simulink model "CSE_SIMULINK_BLOCK_DIAGRAM_NO1"  (R2022b)
settings: Solver=VariableStepAuto  StartTime=0.0  StopTime=10  RelTol=1e-3
undefined symbols (not defined in the file): G1_den, G2_den, G3_den, G_num, H1_den, H2_den, H3_den, H_num, tfden, tfnum
settings Model: Creator=tolen  LastModifiedBy=tolen

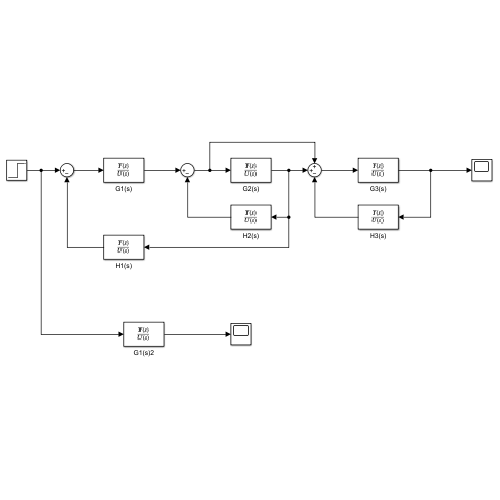
[thumbnail: Simulink's stored preview of the top-level diagram]
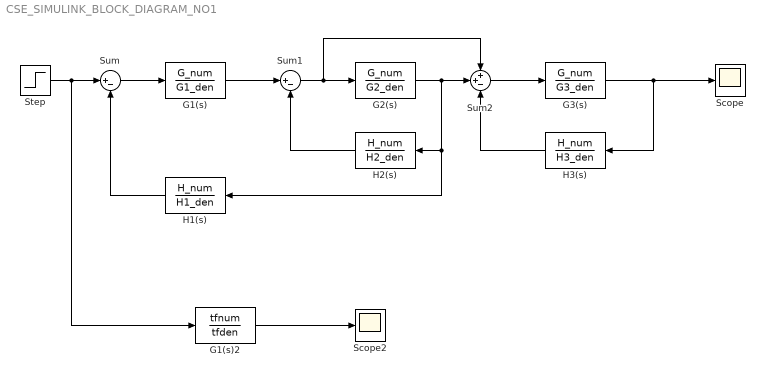
== system CSE_SIMULINK_BLOCK_DIAGRAM_NO1 ==
  G1(s) : TransferFcn  Numerator=G_num  Denominator=G1_den
  G1(s)2 : TransferFcn  Numerator=tfnum  Denominator=tfden
  G2(s) : TransferFcn  Numerator=G_num  Denominator=G2_den
  G3(s) : TransferFcn  Numerator=G_num  Denominator=G3_den
  H1(s) : TransferFcn  Numerator=H_num  Denominator=H1_den
  H2(s) : TransferFcn  Numerator=H_num  Denominator=H2_den
  H3(s) : TransferFcn  Numerator=H_num  Denominator=H3_den
  Scope : Scope
  Scope2 : Scope
  Step : Step  Time=0  SampleTime=0
  Sum : Sum  Inputs=|+-
  Sum1 : Sum  Inputs=|+-
  Sum2 : Sum  Inputs=++-
  wires:
  Sum/1 -> G1(s)/1
  G1(s)/1 -> Sum1/1
  G2(s)/1 -> H2(s)/1, H1(s)/1, Sum2/2
  Sum1/1 -> Sum2/1, G2(s)/1
  Sum2/1 -> G3(s)/1
  G3(s)/1 -> H3(s)/1, Scope/1
  H1(s)/1 -> Sum/2
  H2(s)/1 -> Sum1/2
  H3(s)/1 -> Sum2/3
  G1(s)2/1 -> Scope2/1
  Step/1 -> G1(s)2/1, Sum/1
